simulink model "DC_motor"  (R2014b)
settings: Solver=ode45  StartTime=0.0  StopTime=10.0  RelTol=1e-3
libraries: simulink x1
settings Model: Creator=Asus  LastModifiedBy=Asus

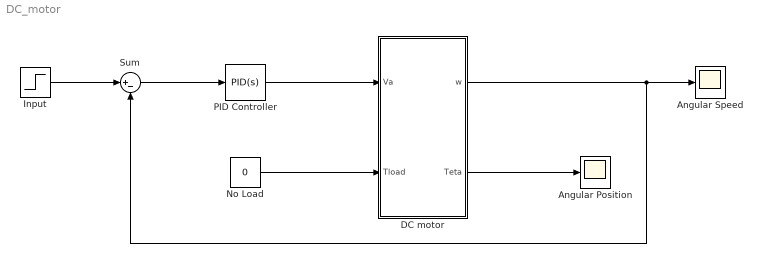
== system DC_motor ==
  Angular Position : Scope
      settings: ShowLegends=on
  Angular Speed : Scope
      settings: ShowLegends=on
  DC motor : Subsystem
  Input : Step  After=10  SampleTime=0
  No Load : Constant  Value=0
  PID Controller : simulink/Continuous/PID Controller  Controller=PID  TimeDomain=Continuous-time  SampleTime=-1  IntegratorMethod=Forward Euler  FilterMethod=Forward Euler  Form=Parallel  P=5  I=0  D=0.4156  N=0  InitialConditionSource=internal  InitialConditionForIntegrator=0  InitialConditionForFilter=0  ExternalReset=none  LimitOutput=off  UpperSaturationLimit=inf  LowerSaturationLimit=-inf  LinearizeAsGain=on  AntiWindupMode=none  Kb=1  TrackingMode=off  Kt=1  PParamMin=[]  PParamMax=[]  IParamMin=[]  IParamMax=[]  DParamMin=[]  DParamMax=[]  NParamMin=[]  NParamMax=[]  KbParamMin=[]  KbParamMax=[]  KtParamMin=[]  KtParamMax=[]  POutMin=[]  POutMax=[]  IOutMin=[]  IOutMax=[]  DOutMin=[]  DOutMax=[]  NOutMin=[]  NOutMax=[]  KbOutMin=[]  KbOutMax=[]  KtOutMin=[]  KtOutMax=[]  IntegratorOutMin=[]  IntegratorOutMax=[]  FilterOutMin=[]  FilterOutMax=[]  SumOutMin=[]  SumOutMax=[]  SumI1OutMin=[]  SumI1OutMax=[]  SumI2OutMin=[]  SumI2OutMax=[]  SumI3OutMin=[]  SumI3OutMax=[]  SumDOutMin=[]  SumDOutMax=[]  SaturationOutMin=[]  SaturationOutMax=[]  IntegratorContinuousStateAttributes=''  IntegratorStateMustResolveToSignalObject=off  IntegratorRTWStateStorageClass=Auto  FilterContinuousStateAttributes=''  FilterStateMustResolveToSignalObject=off  FilterRTWStateStorageClass=Auto  DifferentiatorICPrevScaledInput=0  DifferentiatorOutMin=[]  DifferentiatorOutMax=[]  UseFilter=on
  Sum : Sum  Inputs=|+-
  wires:
  No Load/1 -> DC motor/2(Tload)
  DC motor/1(w) -> Sum/2, Angular Speed/1
  DC motor/2(Teta) -> Angular Position/1
  PID Controller/1 -> DC motor/1(Va)
  Input/1 -> Sum/1
  Sum/1 -> PID Controller/1

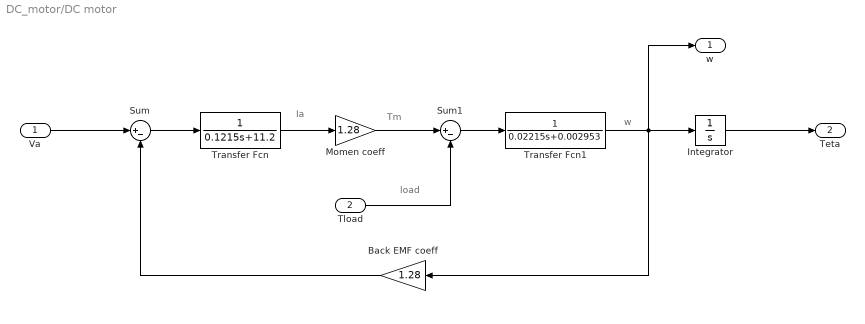
== system DC_motor/DC motor ==
  note: load
  note: Tm
  note: Ia
  note: w
  Va : Inport
  Tload : Inport  Port=2
  Back EMF coeff : Gain  Gain=1.28
  Integrator : Integrator
  Momen coeff : Gain  Gain=1.28
  Sum : Sum  Inputs=|+-
  Sum1 : Sum  Inputs=|+-
  Transfer Fcn : TransferFcn  Denominator=[0.1215 11.2]
  Transfer Fcn1 : TransferFcn  Denominator=[0.02215 0.002953]
  w : Outport
  Teta : Outport  Port=2
  wires:
  Va/1 -> Sum/1
  Sum/1 -> Transfer Fcn/1
  Transfer Fcn/1 -> Momen coeff/1
  Momen coeff/1 -> Sum1/1
  Tload/1 -> Sum1/2
  Sum1/1 -> Transfer Fcn1/1
  Transfer Fcn1/1 -> Back EMF coeff/1, w/1, Integrator/1
  Integrator/1 -> Teta/1
  Back EMF coeff/1 -> Sum/2
